simulink model "parallel_8_cost_function"  (R2022a)
settings: Solver=FixedStepDiscrete  StartTime=0.0  StopTime=10.0  RelTol=1e-3
undefined symbols (not defined in the file or in its folder): f_c
libraries: hdlsllib x1
settings Model: DataTypeOverride=Off  Creator=Andre Merx  LastModifiedBy=Andre Merx
settings SolverCC: AlgebraicLoopSolver=TrustRegion
settings DataIOCC: LimitDataPoints=on  SaveOutput=off  SaveTime=off
settings OptimizationCC: BlockReduction=off  ConditionallyExecuteInputs=off  DefaultParameterBehavior=Inlined  LifeSpan=inf
settings DebuggingCC: AlgebraicLoopMsg=error  SingleTaskRateTransMsg=error  UnconnectedInputMsg=warning  UnconnectedOutputMsg=warning  UnconnectedLineMsg=warning  AllowSymbolicDim=off  StrictBusMsg=ErrorOnBusTreatedAsVector  SFUnexpectedBacktrackingDiag=warning  SFNoUnconditionalDefaultTransitionDiag=warning  SFExecutionAtInitializationDiag=none  SFMachineParentedDataDiag=warning  ArithmeticOperatorsInVariantConditions=warning
settings HardwareCC: ProdBitPerPointer=32  ProdBitPerSizeT=32  ProdBitPerPtrDiffT=32  ProdLargestAtomicFloat=None  ProdIntDivRoundTo=Undefined  ProdEndianess=Unspecified  ProdWordSize=32  ProdHWDeviceType=ASIC/FPGA->ASIC/FPGA  ProdEqTarget=off
settings SFSimCC: SimUseLocalCustomCode=off  CustomCodeUndefinedFunction=UseInterfaceOnly
settings RTWCC: RTWUseLocalCustomCode=off
settings CodeAppCC: StateflowObjectComments=on
settings GRTTargetCC: TargetLangStandard=C89/C90 (ANSI)
settings ConfigComp: CovScope=ReferencedModels  CovMetricSettings=dw  CovSaveCumulativeToWorkspaceVar=on  CovSaveSingleToWorkspaceVar=on  CovExternalEMLEnable=off  CovSFcnEnable=off

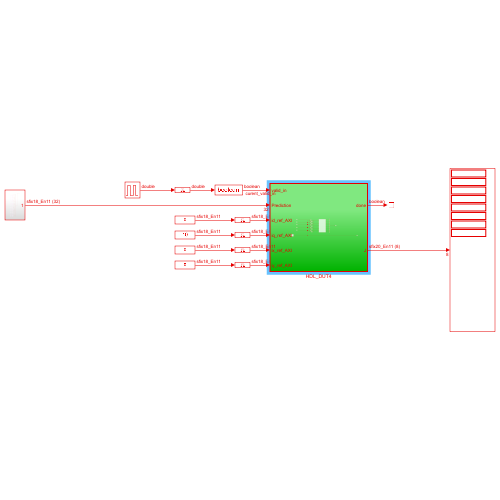
[thumbnail: Simulink's stored preview of the top-level diagram]
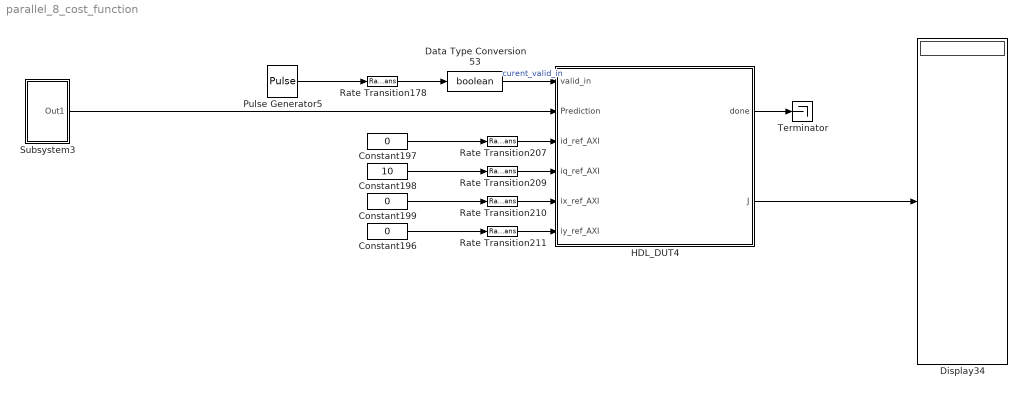
== system parallel_8_cost_function ==
  Constant196 : Constant  Value=0  OutDataTypeStr=fixdt(1,18,11)  SampleTime=-1
  Constant197 : Constant  Value=0  OutDataTypeStr=fixdt(1,18,11)  SampleTime=-1
  Constant198 : Constant  Value=10  OutDataTypeStr=fixdt(1,18,11)  SampleTime=-1
  Constant199 : Constant  Value=0  OutDataTypeStr=fixdt(1,18,11)  SampleTime=-1
  Data Type Conversion53 : DataTypeConversion  OutDataTypeStr=boolean  SaturateOnIntegerOverflow=off  RndMeth=Floor
  Display34 : Display
  HDL_DUT4 : Subsystem  TreatAsAtomicUnit=on
  Pulse Generator5 : DiscretePulseGenerator  PulseType=Time based  Period=1/f_c  PulseWidth=0.1
  Rate Transition{178,207,209..211} (5 alike) : RateTransition  OutPortSampleTime=Rt
  Subsystem3 : Subsystem
  Terminator : Terminator
  wires:
  Rate Transition211/1 -> HDL_DUT4/6(iy_ref_AXI)
  Constant196/1 -> Rate Transition211/1
  Rate Transition210/1 -> HDL_DUT4/5(ix_ref_AXI)
  Rate Transition207/1 -> HDL_DUT4/3(id_ref_AXI)
  Rate Transition209/1 -> HDL_DUT4/4(iq_ref_AXI)
  HDL_DUT4/2(J) -> Display34/1
  Constant198/1 -> Rate Transition209/1
  Constant197/1 -> Rate Transition207/1
  Constant199/1 -> Rate Transition210/1
  Subsystem3/1(Out1) -> HDL_DUT4/2(Prediction)
  HDL_DUT4/1(done) -> Terminator/1
  Rate Transition178/1 -> Data Type Conversion53/1
  Data Type Conversion53/1 -> HDL_DUT4/1(valid_in)  "curent_valid_in"
  Pulse Generator5/1 -> Rate Transition178/1

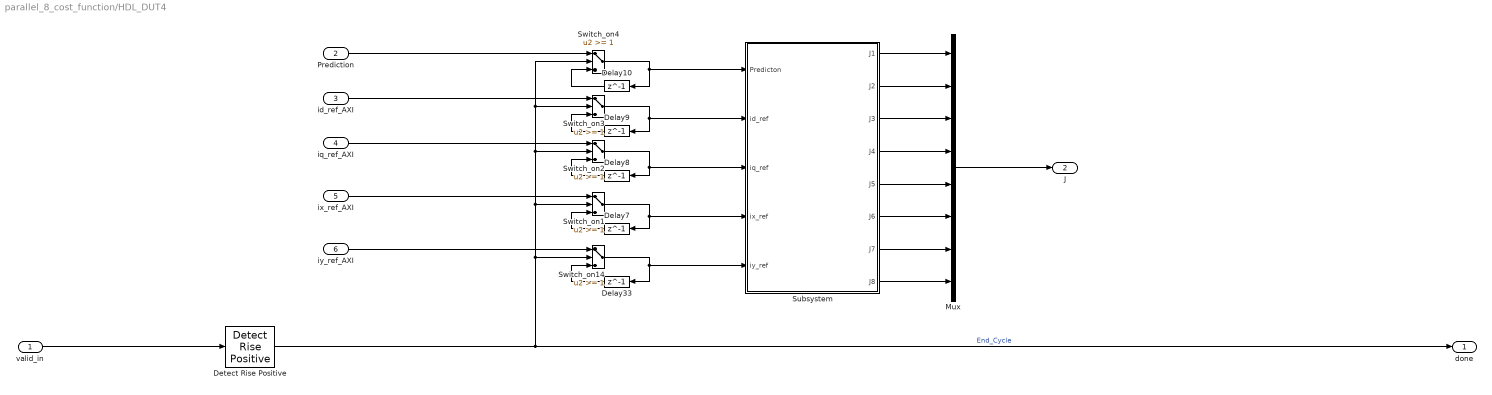
== system parallel_8_cost_function/HDL_DUT4 ==
  valid_in : Inport
  Prediction : Inport  Port=2
  id_ref_AXI : Inport  Port=3
  iq_ref_AXI : Inport  Port=4
  ix_ref_AXI : Inport  Port=5
  iy_ref_AXI : Inport  Port=6
  Delay{7..10,33} (5 alike) : Delay  DelayLength=1
  Detect Rise Positive : hdlsllib/Logic and Bit Operations/Detect Rise Positive  vinit=0  OutDataTypeStr=boolean
      settings: SourceProductBaseCode=SL
  Mux : Mux  Inputs=8
  Subsystem : Subsystem
  Switch_on{1..4,14} (5 alike) : Switch  Threshold=1  OutDataTypeStr=fixdt(1,18,11)  RndMeth=Simplest  SaturateOnIntegerOverflow=off  InputSameDT=off
  done : Outport
  J : Outport  Port=2
  wires:
  iy_ref_AXI/1 -> Switch_on14/1
  Switch_on14/1 -> Delay33/1, Subsystem/5(iy_ref)
  Delay33/1 -> Switch_on14/3
  Delay7/1 -> Switch_on1/3
  ix_ref_AXI/1 -> Switch_on1/1
  Switch_on1/1 -> Subsystem/4(ix_ref), Delay7/1
  Delay8/1 -> Switch_on2/3
  iq_ref_AXI/1 -> Switch_on2/1
  Switch_on2/1 -> Subsystem/3(iq_ref), Delay8/1
  Delay9/1 -> Switch_on3/3
  id_ref_AXI/1 -> Switch_on3/1
  Switch_on3/1 -> Subsystem/2(id_ref), Delay9/1
  Delay10/1 -> Switch_on4/3
  Detect Rise Positive/1 -> done/1, Switch_on4/2, Switch_on3/2, Switch_on2/2, Switch_on1/2, Switch_on14/2  "End_Cycle"
  Prediction/1 -> Switch_on4/1
  Switch_on4/1 -> Delay10/1, Subsystem/1(Predicton)
  Subsystem/1(J1) -> Mux/1
  Subsystem/2(J2) -> Mux/2
  Subsystem/3(J3) -> Mux/3
  Subsystem/4(J4) -> Mux/4
  Subsystem/5(J5) -> Mux/5
  Subsystem/6(J6) -> Mux/6
  Subsystem/7(J7) -> Mux/7
  Subsystem/8(J8) -> Mux/8
  Mux/1 -> J/1
  valid_in/1 -> Detect Rise Positive/1

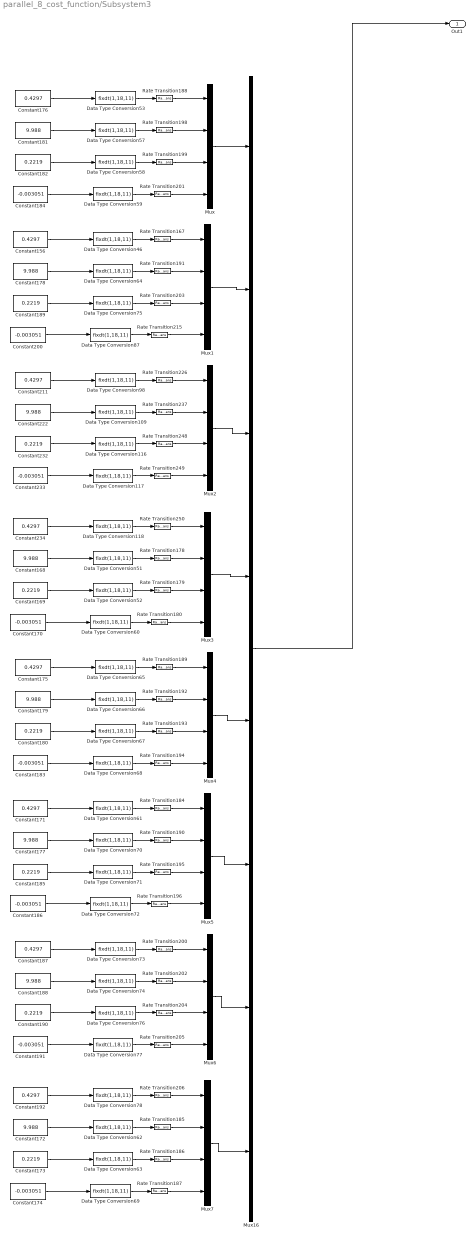
== system parallel_8_cost_function/Subsystem3 ==
  Constant{156,171,175..176,187,192,211,234} (8 alike) : Constant  Value=0.4297
  Constant{168,172,177..179,181,188,222} (8 alike) : Constant  Value=9.988
  Constant{169,173,180,182,185,189..190,232} (8 alike) : Constant  Value=0.2219
  Constant{170,174,183..184,186,191,200,233} (8 alike) : Constant  Value=-0.003051
  Data Type Conversion{46,51..53,57..78,87,98,109,116..118} (32 alike) : DataTypeConversion  OutDataTypeStr=fixdt(1,18,11)  SaturateOnIntegerOverflow=off  RndMeth=Floor
  Mux{,1..7} (8 alike) : Mux
  Mux16 : Mux  Inputs=8
  Rate Transition{167,178..180,184..196,198..206,215,226,237,248..250} (32 alike) : RateTransition  OutPortSampleTime=Rt
  Out1 : Outport
  wires:
  Rate Transition215/1 -> Mux1/4
  Data Type Conversion69/1 -> Rate Transition187/1
  Data Type Conversion71/1 -> Rate Transition195/1
  Data Type Conversion117/1 -> Rate Transition249/1
  Data Type Conversion87/1 -> Rate Transition215/1
  Constant182/1 -> Data Type Conversion58/1
  Rate Transition202/1 -> Mux6/2
  Data Type Conversion70/1 -> Rate Transition190/1
  Constant169/1 -> Data Type Conversion52/1
  Rate Transition178/1 -> Mux3/2
  Constant175/1 -> Data Type Conversion65/1
  Rate Transition193/1 -> Mux4/3
  Data Type Conversion63/1 -> Rate Transition186/1
  Data Type Conversion72/1 -> Rate Transition196/1
  Data Type Conversion75/1 -> Rate Transition203/1
  Rate Transition201/1 -> Mux/4
  Mux7/1 -> Mux16/8
  Rate Transition184/1 -> Mux5/1
  Data Type Conversion65/1 -> Rate Transition189/1
  Data Type Conversion66/1 -> Rate Transition192/1
  Rate Transition190/1 -> Mux5/2
  Rate Transition196/1 -> Mux5/4
  Constant168/1 -> Data Type Conversion51/1
  Constant183/1 -> Data Type Conversion68/1
  Rate Transition187/1 -> Mux7/4
  Constant188/1 -> Data Type Conversion74/1
  Rate Transition189/1 -> Mux4/1
  Mux/1 -> Mux16/1
  Constant172/1 -> Data Type Conversion62/1
  Data Type Conversion61/1 -> Rate Transition184/1
  Data Type Conversion64/1 -> Rate Transition191/1
  Constant187/1 -> Data Type Conversion73/1
  Data Type Conversion74/1 -> Rate Transition202/1
  Rate Transition192/1 -> Mux4/2
  Constant170/1 -> Data Type Conversion60/1
  Data Type Conversion116/1 -> Rate Transition248/1
  Constant176/1 -> Data Type Conversion53/1
  Rate Transition200/1 -> Mux6/1
  Rate Transition250/1 -> Mux3/1
  Constant222/1 -> Data Type Conversion109/1
  Constant184/1 -> Data Type Conversion59/1
  Constant179/1 -> Data Type Conversion66/1
  Mux16/1 -> Out1/1
  Data Type Conversion118/1 -> Rate Transition250/1
  Data Type Conversion53/1 -> Rate Transition188/1
  Rate Transition194/1 -> Mux4/4
  Constant180/1 -> Data Type Conversion67/1
  Constant233/1 -> Data Type Conversion117/1
  Rate Transition167/1 -> Mux1/1
  Constant211/1 -> Data Type Conversion98/1
  Data Type Conversion67/1 -> Rate Transition193/1
  Rate Transition199/1 -> Mux/3
  Rate Transition186/1 -> Mux7/3
  Rate Transition188/1 -> Mux/1
  Constant232/1 -> Data Type Conversion116/1
  Rate Transition226/1 -> Mux2/1
  Data Type Conversion57/1 -> Rate Transition198/1
  Rate Transition237/1 -> Mux2/2
  Constant156/1 -> Data Type Conversion46/1
  Constant181/1 -> Data Type Conversion57/1
  Rate Transition248/1 -> Mux2/3
  Data Type Conversion73/1 -> Rate Transition200/1
  Data Type Conversion60/1 -> Rate Transition180/1
  Constant178/1 -> Data Type Conversion64/1
  Constant173/1 -> Data Type Conversion63/1
  Rate Transition203/1 -> Mux1/3
  Constant177/1 -> Data Type Conversion70/1
  Data Type Conversion109/1 -> Rate Transition237/1
  Constant174/1 -> Data Type Conversion69/1
  Constant185/1 -> Data Type Conversion71/1
  Data Type Conversion59/1 -> Rate Transition201/1
  Rate Transition198/1 -> Mux/2
  Rate Transition180/1 -> Mux3/4
  Constant190/1 -> Data Type Conversion76/1
  Data Type Conversion78/1 -> Rate Transition206/1
  Rate Transition195/1 -> Mux5/3
  Constant186/1 -> Data Type Conversion72/1
  Data Type Conversion62/1 -> Rate Transition185/1
  Rate Transition249/1 -> Mux2/4
  Rate Transition179/1 -> Mux3/3
  Data Type Conversion68/1 -> Rate Transition194/1
  Constant200/1 -> Data Type Conversion87/1
  Data Type Conversion46/1 -> Rate Transition167/1
  Rate Transition205/1 -> Mux6/4
  Data Type Conversion52/1 -> Rate Transition179/1
  Mux6/1 -> Mux16/7
  Data Type Conversion77/1 -> Rate Transition205/1
  Mux1/1 -> Mux16/2
  Mux5/1 -> Mux16/6
  Mux2/1 -> Mux16/3
  Mux3/1 -> Mux16/4
  Constant234/1 -> Data Type Conversion118/1
  Constant171/1 -> Data Type Conversion61/1
  Mux4/1 -> Mux16/5
  Data Type Conversion98/1 -> Rate Transition226/1
  Constant192/1 -> Data Type Conversion78/1
  Rate Transition204/1 -> Mux6/3
  Data Type Conversion58/1 -> Rate Transition199/1
  Constant191/1 -> Data Type Conversion77/1
  Data Type Conversion76/1 -> Rate Transition204/1
  Rate Transition191/1 -> Mux1/2
  Constant189/1 -> Data Type Conversion75/1
  Rate Transition185/1 -> Mux7/2
  Data Type Conversion51/1 -> Rate Transition178/1
  Rate Transition206/1 -> Mux7/1

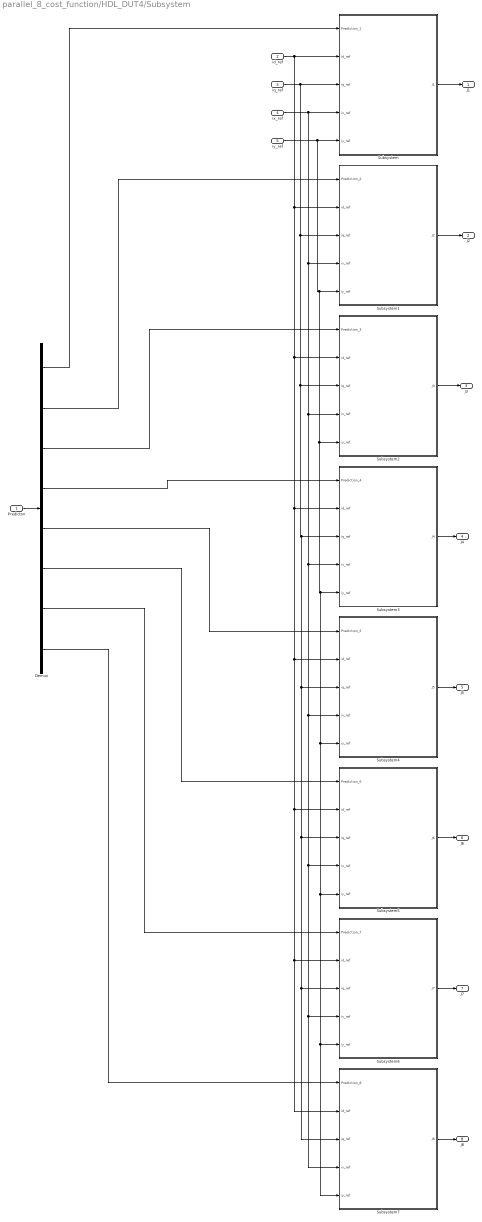
== system parallel_8_cost_function/HDL_DUT4/Subsystem ==
  Predicton : Inport
  id_ref : Inport  Port=2
  iq_ref : Inport  Port=3
  ix_ref : Inport  Port=4
  iy_ref : Inport  Port=5
  Demux : Demux  Outputs=8
  Subsystem : Subsystem
  Subsystem1 : Subsystem
  Subsystem2 : Subsystem
  Subsystem3 : Subsystem
  Subsystem4 : Subsystem
  Subsystem5 : Subsystem
  Subsystem6 : Subsystem
  Subsystem7 : Subsystem
  J1 : Outport
  J2 : Outport  Port=2
  J3 : Outport  Port=3
  J4 : Outport  Port=4
  J5 : Outport  Port=5
  J6 : Outport  Port=6
  J7 : Outport  Port=7
  J8 : Outport  Port=8
  wires:
  Predicton/1 -> Demux/1
  iy_ref/1 -> Subsystem/5(iy_ref), Subsystem7/5(iy_ref), Subsystem6/5(iy_ref), Subsystem5/5(iy_ref), Subsystem4/5(iy_ref), Subsystem3/5(iy_ref), Subsystem2/5(iy_ref), Subsystem1/5(iy_ref)
  ix_ref/1 -> Subsystem/4(ix_ref), Subsystem7/4(ix_ref), Subsystem6/4(ix_ref), Subsystem5/4(ix_ref), Subsystem4/4(ix_ref), Subsystem3/4(ix_ref), Subsystem2/4(ix_ref), Subsystem1/4(ix_ref)
  iq_ref/1 -> Subsystem/3(iq_ref), Subsystem7/3(iq_ref), Subsystem6/3(iq_ref), Subsystem5/3(iq_ref), Subsystem4/3(iq_ref), Subsystem3/3(iq_ref), Subsystem2/3(iq_ref), Subsystem1/3(iq_ref)
  id_ref/1 -> Subsystem7/2(id_ref), Subsystem6/2(id_ref), Subsystem5/2(id_ref), Subsystem4/2(id_ref), Subsystem3/2(id_ref), Subsystem2/2(id_ref), Subsystem1/2(id_ref), Subsystem/2(id_ref)
  Demux/1 -> Subsystem/1(Prediction_1)
  Demux/2 -> Subsystem1/1(Prediction_2)
  Demux/3 -> Subsystem2/1(Prediction_3)
  Demux/4 -> Subsystem3/1(Prediction_4)
  Demux/5 -> Subsystem4/1(Prediction_5)
  Demux/6 -> Subsystem5/1(Prediction_6)
  Demux/7 -> Subsystem6/1(Prediction_7)
  Demux/8 -> Subsystem7/1(Prediction_8)
  Subsystem/1(J1) -> J1/1
  Subsystem1/1(J2) -> J2/1
  Subsystem2/1(J3) -> J3/1
  Subsystem3/1(J4) -> J4/1
  Subsystem4/1(J5) -> J5/1
  Subsystem5/1(J6) -> J6/1
  Subsystem6/1(J7) -> J7/1
  Subsystem7/1(J8) -> J8/1

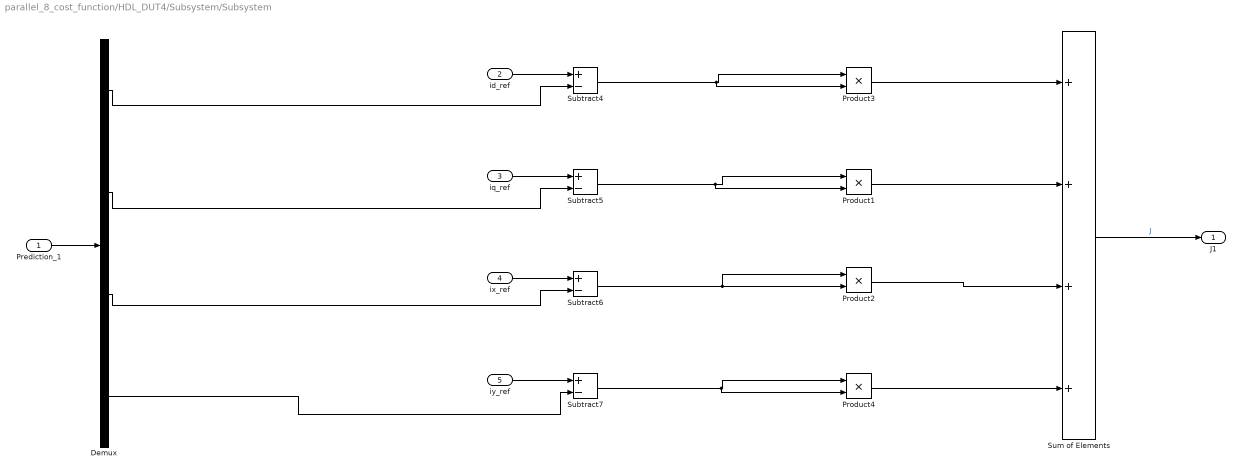
== system parallel_8_cost_function/HDL_DUT4/Subsystem/Subsystem ==
  Prediction_1 : Inport
  id_ref : Inport  Port=2
  iq_ref : Inport  Port=3
  ix_ref : Inport  Port=4
  iy_ref : Inport  Port=5
  Demux : Demux
  Product{1..4} (4 alike) : Product  OutDataTypeStr=fixdt(1,20,11)
  Subtract{4..7} (4 alike) : Sum  Inputs=+-  OutDataTypeStr=fixdt(1,20,11)
  Sum of Elements : Sum  Inputs=++++  OutDataTypeStr=fixdt(1,20,11)
  J1 : Outport
  wires:
  Prediction_1/1 -> Demux/1
  iy_ref/1 -> Subtract7/1
  Demux/3 -> Subtract6/2
  Sum of Elements/1 -> J1/1  "J"
  iq_ref/1 -> Subtract5/1
  id_ref/1 -> Subtract4/1
  Demux/2 -> Subtract5/2
  ix_ref/1 -> Subtract6/1
  Demux/4 -> Subtract7/2
  Demux/1 -> Subtract4/2
  Product3/1 -> Sum of Elements/1
  Product1/1 -> Sum of Elements/2
  Product2/1 -> Sum of Elements/3
  Product4/1 -> Sum of Elements/4
  Subtract4/1 -> Product3/2, Product3/1
  Subtract5/1 -> Product1/2, Product1/1
  Subtract6/1 -> Product2/2, Product2/1
  Subtract7/1 -> Product4/2, Product4/1

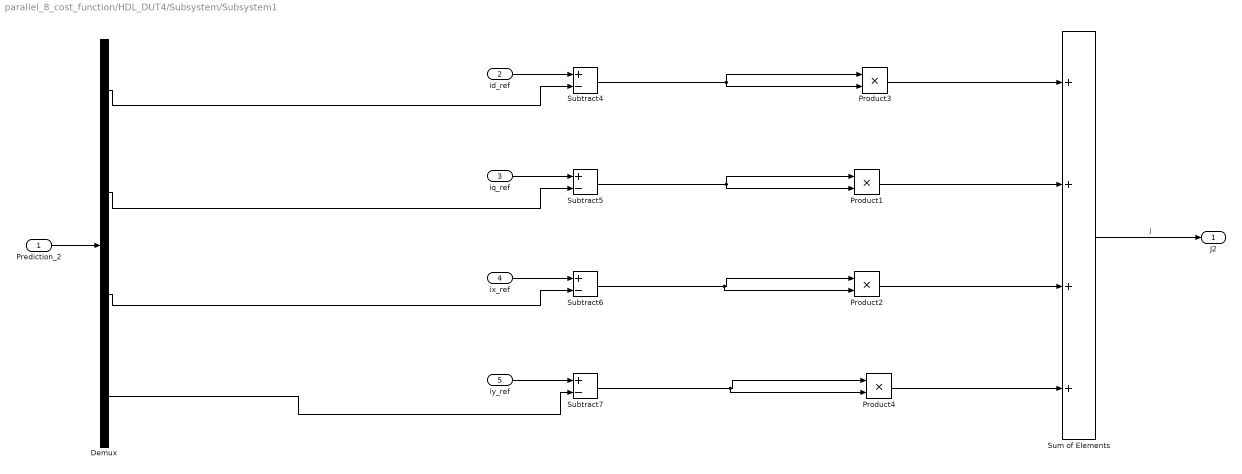
== system parallel_8_cost_function/HDL_DUT4/Subsystem/Subsystem1 ==
  Prediction_2 : Inport
  id_ref : Inport  Port=2
  iq_ref : Inport  Port=3
  ix_ref : Inport  Port=4
  iy_ref : Inport  Port=5
  Demux : Demux
  Product{1..4} (4 alike) : Product  OutDataTypeStr=fixdt(1,20,11)
  Subtract{4..7} (4 alike) : Sum  Inputs=+-  OutDataTypeStr=fixdt(1,20,11)
  Sum of Elements : Sum  Inputs=++++  OutDataTypeStr=fixdt(1,20,11)
  J2 : Outport
  wires:
  Prediction_2/1 -> Demux/1
  iy_ref/1 -> Subtract7/1
  Demux/3 -> Subtract6/2
  Sum of Elements/1 -> J2/1  "J"
  iq_ref/1 -> Subtract5/1
  id_ref/1 -> Subtract4/1
  Demux/2 -> Subtract5/2
  ix_ref/1 -> Subtract6/1
  Demux/4 -> Subtract7/2
  Demux/1 -> Subtract4/2
  Product3/1 -> Sum of Elements/1
  Product1/1 -> Sum of Elements/2
  Product2/1 -> Sum of Elements/3
  Product4/1 -> Sum of Elements/4
  Subtract4/1 -> Product3/2, Product3/1
  Subtract5/1 -> Product1/2, Product1/1
  Subtract6/1 -> Product2/2, Product2/1
  Subtract7/1 -> Product4/2, Product4/1

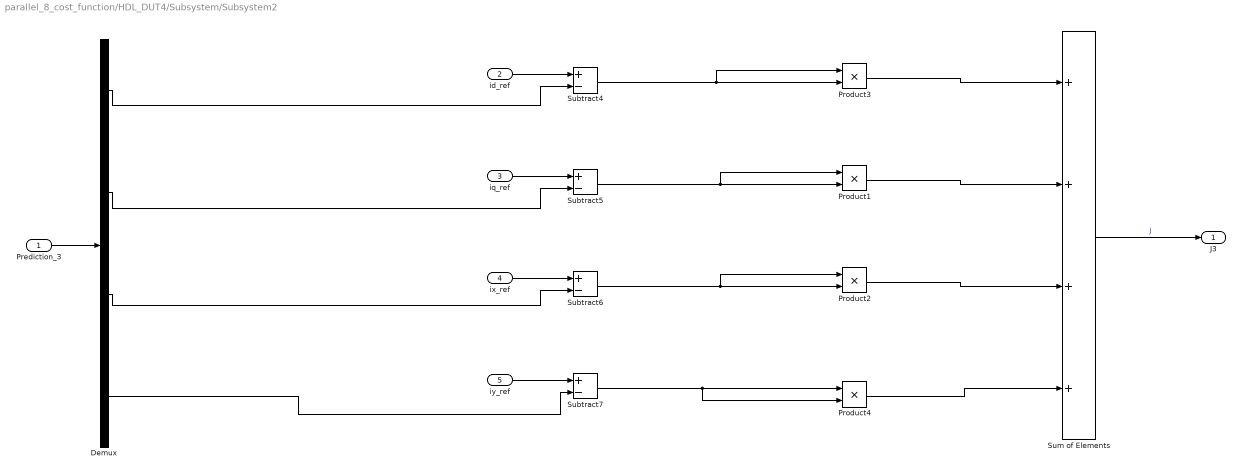
== system parallel_8_cost_function/HDL_DUT4/Subsystem/Subsystem2 ==
  Prediction_3 : Inport
  id_ref : Inport  Port=2
  iq_ref : Inport  Port=3
  ix_ref : Inport  Port=4
  iy_ref : Inport  Port=5
  Demux : Demux
  Product{1..4} (4 alike) : Product  OutDataTypeStr=fixdt(1,20,11)
  Subtract{4..7} (4 alike) : Sum  Inputs=+-  OutDataTypeStr=fixdt(1,20,11)
  Sum of Elements : Sum  Inputs=++++  OutDataTypeStr=fixdt(1,20,11)
  J3 : Outport
  wires:
  Prediction_3/1 -> Demux/1
  iy_ref/1 -> Subtract7/1
  Demux/3 -> Subtract6/2
  Sum of Elements/1 -> J3/1  "J"
  iq_ref/1 -> Subtract5/1
  id_ref/1 -> Subtract4/1
  Demux/2 -> Subtract5/2
  ix_ref/1 -> Subtract6/1
  Demux/4 -> Subtract7/2
  Demux/1 -> Subtract4/2
  Product3/1 -> Sum of Elements/1
  Product1/1 -> Sum of Elements/2
  Product2/1 -> Sum of Elements/3
  Product4/1 -> Sum of Elements/4
  Subtract4/1 -> Product3/2, Product3/1
  Subtract5/1 -> Product1/2, Product1/1
  Subtract6/1 -> Product2/2, Product2/1
  Subtract7/1 -> Product4/2, Product4/1

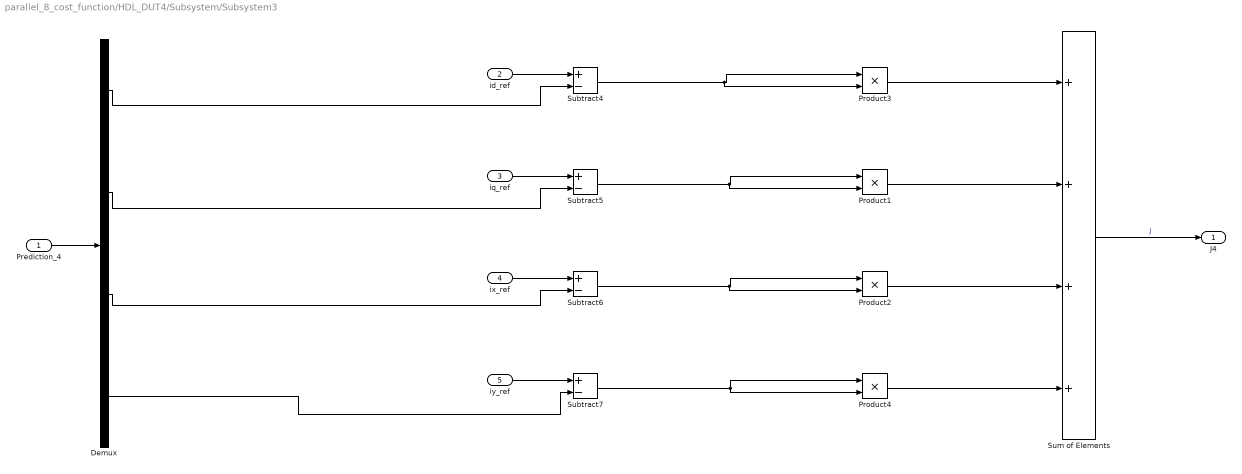
== system parallel_8_cost_function/HDL_DUT4/Subsystem/Subsystem3 ==
  Prediction_4 : Inport
  id_ref : Inport  Port=2
  iq_ref : Inport  Port=3
  ix_ref : Inport  Port=4
  iy_ref : Inport  Port=5
  Demux : Demux
  Product{1..4} (4 alike) : Product  OutDataTypeStr=fixdt(1,20,11)
  Subtract{4..7} (4 alike) : Sum  Inputs=+-  OutDataTypeStr=fixdt(1,20,11)
  Sum of Elements : Sum  Inputs=++++  OutDataTypeStr=fixdt(1,20,11)
  J4 : Outport
  wires:
  Prediction_4/1 -> Demux/1
  iy_ref/1 -> Subtract7/1
  Demux/3 -> Subtract6/2
  Sum of Elements/1 -> J4/1  "J"
  iq_ref/1 -> Subtract5/1
  id_ref/1 -> Subtract4/1
  Demux/2 -> Subtract5/2
  ix_ref/1 -> Subtract6/1
  Demux/4 -> Subtract7/2
  Demux/1 -> Subtract4/2
  Product3/1 -> Sum of Elements/1
  Product1/1 -> Sum of Elements/2
  Product2/1 -> Sum of Elements/3
  Product4/1 -> Sum of Elements/4
  Subtract4/1 -> Product3/2, Product3/1
  Subtract5/1 -> Product1/2, Product1/1
  Subtract6/1 -> Product2/2, Product2/1
  Subtract7/1 -> Product4/2, Product4/1

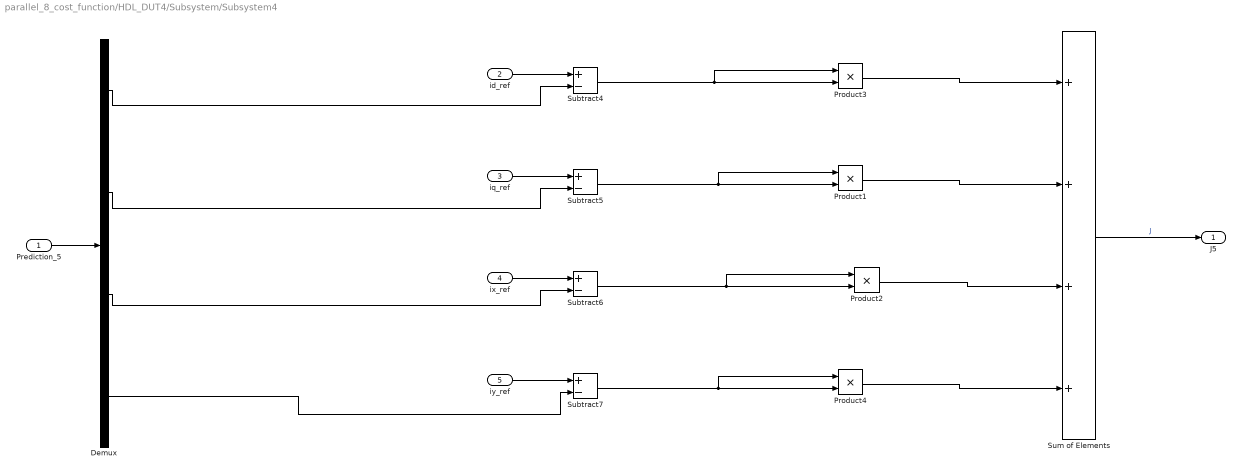
== system parallel_8_cost_function/HDL_DUT4/Subsystem/Subsystem4 ==
  Prediction_5 : Inport
  id_ref : Inport  Port=2
  iq_ref : Inport  Port=3
  ix_ref : Inport  Port=4
  iy_ref : Inport  Port=5
  Demux : Demux
  Product{1..4} (4 alike) : Product  OutDataTypeStr=fixdt(1,20,11)
  Subtract{4..7} (4 alike) : Sum  Inputs=+-  OutDataTypeStr=fixdt(1,20,11)
  Sum of Elements : Sum  Inputs=++++  OutDataTypeStr=fixdt(1,20,11)
  J5 : Outport
  wires:
  Prediction_5/1 -> Demux/1
  iy_ref/1 -> Subtract7/1
  Demux/3 -> Subtract6/2
  Sum of Elements/1 -> J5/1  "J"
  iq_ref/1 -> Subtract5/1
  id_ref/1 -> Subtract4/1
  Demux/2 -> Subtract5/2
  ix_ref/1 -> Subtract6/1
  Demux/4 -> Subtract7/2
  Demux/1 -> Subtract4/2
  Product3/1 -> Sum of Elements/1
  Product1/1 -> Sum of Elements/2
  Product2/1 -> Sum of Elements/3
  Product4/1 -> Sum of Elements/4
  Subtract4/1 -> Product3/1, Product3/2
  Subtract5/1 -> Product1/2, Product1/1
  Subtract6/1 -> Product2/2, Product2/1
  Subtract7/1 -> Product4/2, Product4/1

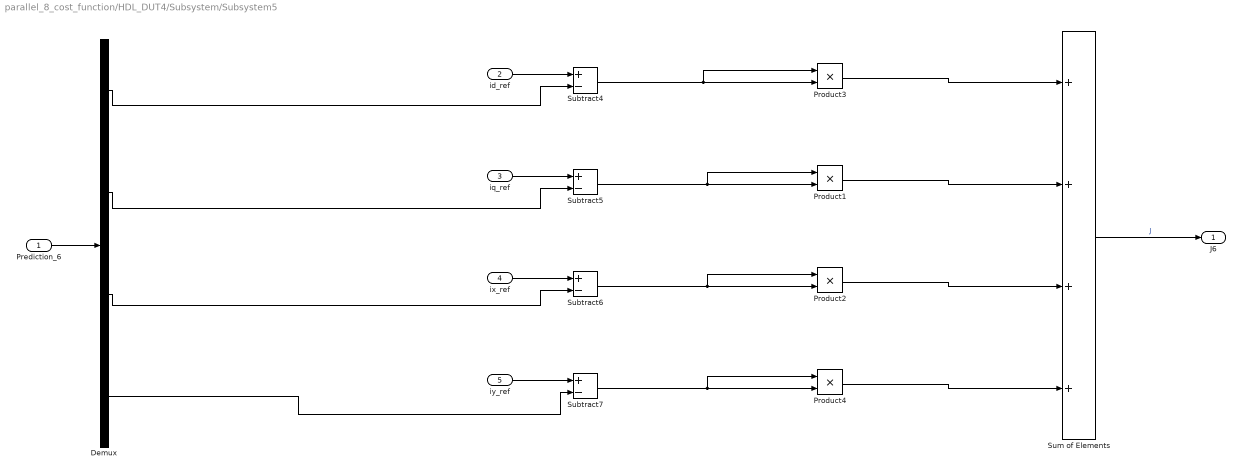
== system parallel_8_cost_function/HDL_DUT4/Subsystem/Subsystem5 ==
  Prediction_6 : Inport
  id_ref : Inport  Port=2
  iq_ref : Inport  Port=3
  ix_ref : Inport  Port=4
  iy_ref : Inport  Port=5
  Demux : Demux
  Product{1..4} (4 alike) : Product  OutDataTypeStr=fixdt(1,20,11)
  Subtract{4..7} (4 alike) : Sum  Inputs=+-  OutDataTypeStr=fixdt(1,20,11)
  Sum of Elements : Sum  Inputs=++++  OutDataTypeStr=fixdt(1,20,11)
  J6 : Outport
  wires:
  Prediction_6/1 -> Demux/1
  iy_ref/1 -> Subtract7/1
  Demux/3 -> Subtract6/2
  Sum of Elements/1 -> J6/1  "J"
  iq_ref/1 -> Subtract5/1
  id_ref/1 -> Subtract4/1
  Demux/2 -> Subtract5/2
  ix_ref/1 -> Subtract6/1
  Demux/4 -> Subtract7/2
  Demux/1 -> Subtract4/2
  Product3/1 -> Sum of Elements/1
  Product1/1 -> Sum of Elements/2
  Product2/1 -> Sum of Elements/3
  Product4/1 -> Sum of Elements/4
  Subtract4/1 -> Product3/2, Product3/1
  Subtract5/1 -> Product1/1, Product1/2
  Subtract6/1 -> Product2/2, Product2/1
  Subtract7/1 -> Product4/2, Product4/1

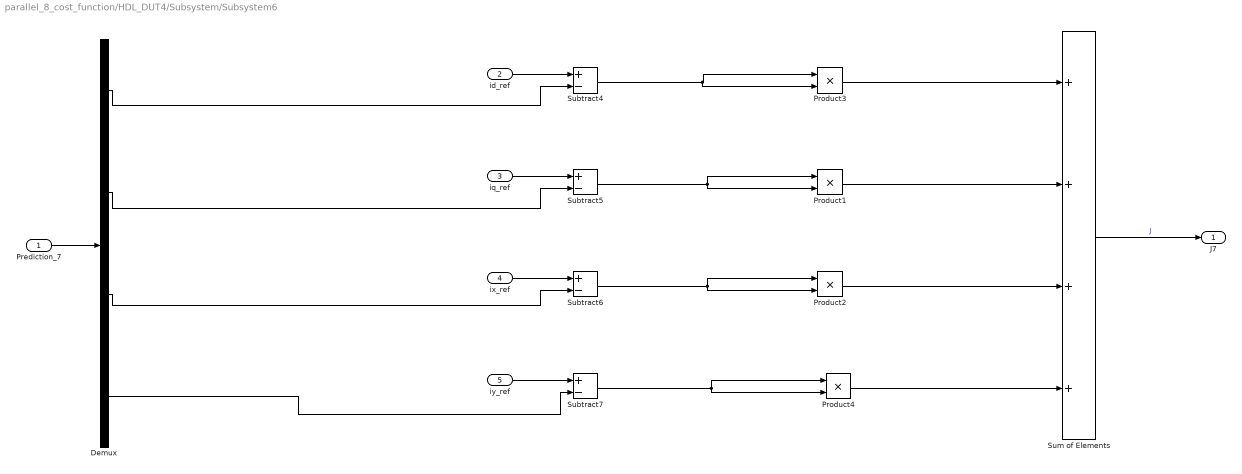
== system parallel_8_cost_function/HDL_DUT4/Subsystem/Subsystem6 ==
  Prediction_7 : Inport
  id_ref : Inport  Port=2
  iq_ref : Inport  Port=3
  ix_ref : Inport  Port=4
  iy_ref : Inport  Port=5
  Demux : Demux
  Product{1..4} (4 alike) : Product  OutDataTypeStr=fixdt(1,20,11)
  Subtract{4..7} (4 alike) : Sum  Inputs=+-  OutDataTypeStr=fixdt(1,20,11)
  Sum of Elements : Sum  Inputs=++++  OutDataTypeStr=fixdt(1,20,11)
  J7 : Outport
  wires:
  Prediction_7/1 -> Demux/1
  iy_ref/1 -> Subtract7/1
  Demux/3 -> Subtract6/2
  Sum of Elements/1 -> J7/1  "J"
  iq_ref/1 -> Subtract5/1
  id_ref/1 -> Subtract4/1
  Demux/2 -> Subtract5/2
  ix_ref/1 -> Subtract6/1
  Demux/4 -> Subtract7/2
  Demux/1 -> Subtract4/2
  Product3/1 -> Sum of Elements/1
  Product1/1 -> Sum of Elements/2
  Product2/1 -> Sum of Elements/3
  Product4/1 -> Sum of Elements/4
  Subtract4/1 -> Product3/2, Product3/1
  Subtract5/1 -> Product1/2, Product1/1
  Subtract6/1 -> Product2/2, Product2/1
  Subtract7/1 -> Product4/2, Product4/1

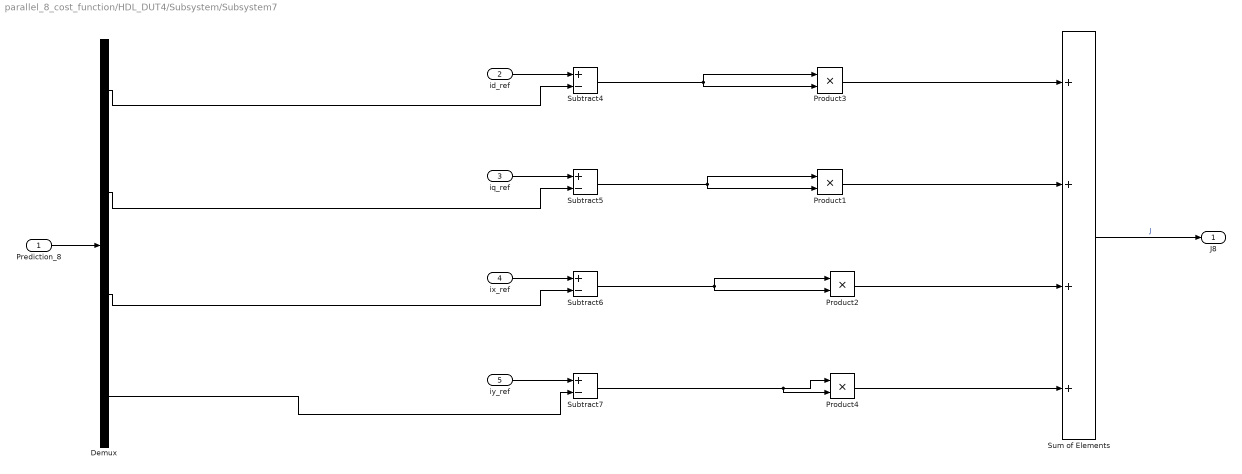
== system parallel_8_cost_function/HDL_DUT4/Subsystem/Subsystem7 ==
  Prediction_8 : Inport
  id_ref : Inport  Port=2
  iq_ref : Inport  Port=3
  ix_ref : Inport  Port=4
  iy_ref : Inport  Port=5
  Demux : Demux
  Product{1..4} (4 alike) : Product  OutDataTypeStr=fixdt(1,20,11)
  Subtract{4..7} (4 alike) : Sum  Inputs=+-  OutDataTypeStr=fixdt(1,20,11)
  Sum of Elements : Sum  Inputs=++++  OutDataTypeStr=fixdt(1,20,11)
  J8 : Outport
  wires:
  Prediction_8/1 -> Demux/1
  iy_ref/1 -> Subtract7/1
  Demux/3 -> Subtract6/2
  Sum of Elements/1 -> J8/1  "J"
  iq_ref/1 -> Subtract5/1
  id_ref/1 -> Subtract4/1
  Demux/2 -> Subtract5/2
  ix_ref/1 -> Subtract6/1
  Demux/4 -> Subtract7/2
  Demux/1 -> Subtract4/2
  Product3/1 -> Sum of Elements/1
  Product1/1 -> Sum of Elements/2
  Product2/1 -> Sum of Elements/3
  Product4/1 -> Sum of Elements/4
  Subtract4/1 -> Product3/1, Product3/2
  Subtract5/1 -> Product1/1, Product1/2
  Subtract6/1 -> Product2/1, Product2/2
  Subtract7/1 -> Product4/2, Product4/1
